simulink model "KUKA_Linear"  (R2020b)
settings: Solver=VariableStepAuto  StartTime=0.0  StopTime=200  RelTol=1e-3
(part 3 of 3)

== matlab function KUKA_Linear/Subsystem/Jacobian//Jacobian_dot//X_dot//X_ddot ==
  data: J output; q1 input; J_dot output; q1_dot input; q2 input; q2_dot input; q3 input; q3_dot input; q4 input; q4_dot input; q1_ddot input; q2_ddot input; q3_ddot input; X_dot output; X_ddot output; q4_ddot input; Theta_dot output; Theta_ddot output
function [J, J_dot, X_dot, X_ddot, Theta_dot, Theta_ddot] = fcn(q1, q1_dot, q2, q2_dot, q3, q3_dot, q4, q4_dot, q1_ddot, q2_ddot, q3_ddot, q4_ddot)

d3 = 0.4;
d5 = 0.39;

%#codegen
theta_1 = q1;
theta_2 = q2;
theta_3 = q3;
theta_4 = q4;

theta_1_dot = q1_dot;
theta_2_dot = q2_dot;
theta_3_dot = q3_dot;
theta_4_dot = q1_dot;

j1 = [  d3*sin(theta_1)*sin(theta_2) - d5*(sin(theta_4)*(cos(theta_1)*sin(theta_3) + cos(theta_2)*cos(theta_3)*sin(theta_1)) - cos(theta_4)*sin(theta_1)*sin(theta_2)), - d5*(cos(theta_1)*cos(theta_2)*cos(theta_4) + cos(theta_1)*cos(theta_3)*sin(theta_2)*sin(theta_4)) - d3*cos(theta_1)*cos(theta_2), -d5*sin(theta_4)*(cos(theta_3)*sin(theta_1) + cos(theta_1)*cos(theta_2)*sin(theta_3)), -d5*(cos(theta_4)*(sin(theta_1)*sin(theta_3) - cos(theta_1)*cos(theta_2)*cos(theta_3)) - cos(theta_1)*sin(theta_2)*sin(theta_4))];
j2 = [- d5*(sin(theta_4)*(sin(theta_1)*sin(theta_3) - cos(theta_1)*cos(theta_2)*cos(theta_3)) + cos(theta_1)*cos(theta_4)*sin(theta_2)) - d3*cos(theta_1)*sin(theta_2), - d5*(cos(theta_2)*cos(theta_4)*sin(theta_1) + cos(theta_3)*sin(theta_1)*sin(theta_2)*sin(theta_4)) - d3*cos(theta_2)*sin(theta_1),  d5*sin(theta_4)*(cos(theta_1)*cos(theta_3) - cos(theta_2)*sin(theta_1)*sin(theta_3)),  d5*(cos(theta_4)*(cos(theta_1)*sin(theta_3) + cos(theta_2)*cos(theta_3)*sin(theta_1)) + sin(theta_1)*sin(theta_2)*sin(theta_4))];
j3 = [                                                                                                                                                               0,                                        - d5*(cos(theta_4)*sin(theta_2) - cos(theta_2)*cos(theta_3)*sin(theta_4)) - d3*sin(theta_2),                                            -d5*sin(theta_2)*sin(theta_3)*sin(theta_4),                                                         -d5*(cos(theta_2)*sin(theta_4) - cos(theta_3)*cos(theta_4)*sin(theta_2))];

Jv = [j1;j2;j3];

j1_dot = [  theta_1_dot*(d5*(sin(theta_4)*(sin(theta_1)*sin(theta_3) - cos(theta_1)*cos(theta_2)*cos(theta_3)) + cos(theta_1)*cos(theta_4)*sin(theta_2)) + d3*cos(theta_1)*sin(theta_2)) + theta_2_dot*(d5*(cos(theta_2)*cos(theta_4)*sin(theta_1) + cos(theta_3)*sin(theta_1)*sin(theta_2)*sin(theta_4)) + d3*cos(theta_2)*sin(theta_1)) - d5*theta_4_dot*(cos(theta_4)*(cos(theta_1)*sin(theta_3) + cos(theta_2)*cos(theta_3)*sin(theta_1)) + sin(theta_1)*sin(theta_2)*sin(theta_4)) - d5*theta_3_dot*sin(theta_4)*(cos(theta_1)*cos(theta_3) - cos(theta_2)*sin(theta_1)*sin(theta_3)), theta_2_dot*(d5*(cos(theta_1)*cos(theta_4)*sin(theta_2) - cos(theta_1)*cos(theta_2)*cos(theta_3)*sin(theta_4)) + d3*cos(theta_1)*sin(theta_2)) + theta_1_dot*(d5*(cos(theta_2)*cos(theta_4)*sin(theta_1) + cos(theta_3)*sin(theta_1)*sin(theta_2)*sin(theta_4)) + d3*cos(theta_2)*sin(theta_1)) + d5*theta_4_dot*(cos(theta_1)*cos(theta_2)*sin(theta_4) - cos(theta_1)*cos(theta_3)*cos(theta_4)*sin(theta_2)) + d5*theta_3_dot*cos(theta_1)*sin(theta_2)*sin(theta_3)*sin(theta_4), d5*theta_3_dot*sin(theta_4)*(sin(theta_1)*sin(theta_3) - cos(theta_1)*cos(theta_2)*cos(theta_3)) - d5*theta_1_dot*sin(theta_4)*(cos(theta_1)*cos(theta_3) - cos(theta_2)*sin(theta_1)*sin(theta_3)) - d5*theta_4_dot*cos(theta_4)*(cos(theta_3)*sin(theta_1) + cos(theta_1)*cos(theta_2)*sin(theta_3)) + d5*theta_2_dot*cos(theta_1)*sin(theta_2)*sin(theta_3)*sin(theta_4), d5*theta_4_dot*(sin(theta_4)*(sin(theta_1)*sin(theta_3) - cos(theta_1)*cos(theta_2)*cos(theta_3)) + cos(theta_1)*cos(theta_4)*sin(theta_2)) - d5*theta_1_dot*(cos(theta_4)*(cos(theta_1)*sin(theta_3) + cos(theta_2)*cos(theta_3)*sin(theta_1)) + sin(theta_1)*sin(theta_2)*sin(theta_4)) + d5*theta_2_dot*(cos(theta_1)*cos(theta_2)*sin(theta_4) - cos(theta_1)*cos(theta_3)*cos(theta_4)*sin(theta_2)) - d5*theta_3_dot*cos(theta_4)*(cos(theta_3)*sin(theta_1) + cos(theta_1)*cos(theta_2)*sin(theta_3))                                                                                                                                                                                                                                                                                                                                                                                                                                                                                                  ];
j2_dot = [- theta_2_dot*(d5*(cos(theta_1)*cos(theta_2)*cos(theta_4) + cos(theta_1)*cos(theta_3)*sin(theta_2)*sin(theta_4)) + d3*cos(theta_1)*cos(theta_2)) - theta_1_dot*(d5*(sin(theta_4)*(cos(theta_1)*sin(theta_3) + cos(theta_2)*cos(theta_3)*sin(theta_1)) - cos(theta_4)*sin(theta_1)*sin(theta_2)) - d3*sin(theta_1)*sin(theta_2)) - d5*theta_4_dot*(cos(theta_4)*(sin(theta_1)*sin(theta_3) - cos(theta_1)*cos(theta_2)*cos(theta_3)) - cos(theta_1)*sin(theta_2)*sin(theta_4)) - d5*theta_3_dot*sin(theta_4)*(cos(theta_3)*sin(theta_1) + cos(theta_1)*cos(theta_2)*sin(theta_3)), theta_2_dot*(d5*(cos(theta_4)*sin(theta_1)*sin(theta_2) - cos(theta_2)*cos(theta_3)*sin(theta_1)*sin(theta_4)) + d3*sin(theta_1)*sin(theta_2)) - theta_1_dot*(d5*(cos(theta_1)*cos(theta_2)*cos(theta_4) + cos(theta_1)*cos(theta_3)*sin(theta_2)*sin(theta_4)) + d3*cos(theta_1)*cos(theta_2)) + d5*theta_4_dot*(cos(theta_2)*sin(theta_1)*sin(theta_4) - cos(theta_3)*cos(theta_4)*sin(theta_1)*sin(theta_2)) + d5*theta_3_dot*sin(theta_1)*sin(theta_2)*sin(theta_3)*sin(theta_4), d5*theta_4_dot*cos(theta_4)*(cos(theta_1)*cos(theta_3) - cos(theta_2)*sin(theta_1)*sin(theta_3)) - d5*theta_1_dot*sin(theta_4)*(cos(theta_3)*sin(theta_1) + cos(theta_1)*cos(theta_2)*sin(theta_3)) - d5*theta_3_dot*sin(theta_4)*(cos(theta_1)*sin(theta_3) + cos(theta_2)*cos(theta_3)*sin(theta_1)) + d5*theta_2_dot*sin(theta_1)*sin(theta_2)*sin(theta_3)*sin(theta_4), d5*theta_2_dot*(cos(theta_2)*sin(theta_1)*sin(theta_4) - cos(theta_3)*cos(theta_4)*sin(theta_1)*sin(theta_2)) - d5*theta_4_dot*(sin(theta_4)*(cos(theta_1)*sin(theta_3) + cos(theta_2)*cos(theta_3)*sin(theta_1)) - cos(theta_4)*sin(theta_1)*sin(theta_2)) - d5*theta_1_dot*(cos(theta_4)*(sin(theta_1)*sin(theta_3) - cos(theta_1)*cos(theta_2)*cos(theta_3)) - cos(theta_1)*sin(theta_2)*sin(theta_4)) + d5*theta_3_dot*cos(theta_4)*(cos(theta_1)*cos(theta_3) - cos(theta_2)*sin(theta_1)*sin(theta_3))                                                                                                                                                                                                                                                                                                                                                                                                                                                                                                  ];
j3_dot = [                                                                                                                                                                                                                                                                                                                                                                                                                                                                                                                                                                               0,                                                                                                                                                                                                                                d5*theta_4_dot*(sin(theta_2)*sin(theta_4) + cos(theta_2)*cos(theta_3)*cos(theta_4)) - theta_2_dot*(d5*(cos(theta_2)*cos(theta_4) + cos(theta_3)*sin(theta_2)*sin(theta_4)) + d3*cos(theta_2)) - d5*theta_3_dot*cos(theta_2)*sin(theta_3)*sin(theta_4),                                                                                                                                                                                                     - d5*theta_2_dot*cos(theta_2)*sin(theta_3)*sin(theta_4) - d5*theta_3_dot*cos(theta_3)*sin(theta_2)*sin(theta_4) - d5*theta_4_dot*cos(theta_4)*sin(theta_2)*sin(theta_3),                                                                                                                                                                                                                                                                            d5*theta_2_dot*(sin(theta_2)*sin(theta_4) + cos(theta_2)*cos(theta_3)*cos(theta_4)) - d5*theta_4_dot*(cos(theta_2)*cos(theta_4) + cos(theta_3)*sin(theta_2)*sin(theta_4)) - d5*theta_3_dot*cos(theta_4)*sin(theta_2)*sin(theta_3)                                                                                                                                                                                                                                                                                                                                                                                                                                                                                                  ];

Jv_dot = [j1_dot;j2_dot;j3_dot];

X_dot = Jv*[q1_dot ; q2_dot ; q3_dot; q4_dot];
X_ddot = Jv_dot*[q1_dot ; q2_dot ; q3_dot; q4_dot] + Jv*[q1_ddot ; q2_ddot ; q3_ddot; q4_ddot];

jw1 = [                                                                                                                                                               0,                                                                                                                       sin(theta_1),                                                            -cos(theta_1)*sin(theta_2),                                                             - cos(theta_3)*sin(theta_1) - cos(theta_1)*cos(theta_2)*sin(theta_3)];
jw2 = [                                                                                                                                                               0,                                                                                                                      -cos(theta_1),                                                            -sin(theta_1)*sin(theta_2),                                                               cos(theta_1)*cos(theta_3) - cos(theta_2)*sin(theta_1)*sin(theta_3)];
jw3 = [                                                                                                                                                               1,                                                                                                                                  0,                                                                          cos(theta_2),                                                                                                       -sin(theta_2)*sin(theta_3)];

Jw = [jw1;jw2;jw3];

jw1_dot = [                                                                                                                                                                                                                                                                                                                                                                                                                                                                                                                                                                               0,                                                                                                                                                                                                                                                                                                                                                                                                                                                             theta_1_dot*cos(theta_1),                                                                                                                                                                                                                                                                                               theta_1_dot*sin(theta_1)*sin(theta_2) - theta_2_dot*cos(theta_1)*cos(theta_2),                                                                                                                                                                                                                                                                                     theta_3_dot*(sin(theta_1)*sin(theta_3) - cos(theta_1)*cos(theta_2)*cos(theta_3)) - theta_1_dot*(cos(theta_1)*cos(theta_3) - cos(theta_2)*sin(theta_1)*sin(theta_3)) + theta_2_dot*cos(theta_1)*sin(theta_2)*sin(theta_3)];
jw2_dot = [                                                                                                                                                                                                                                                                                                                                                                                                                                                                                                                                                                               0,                                                                                                                                                                                                                                                                                                                                                                                                                                                             theta_1_dot*sin(theta_1),                                                                                                                                                                                                                                                                                             - theta_1_dot*cos(theta_1)*sin(theta_2) - theta_2_dot*cos(theta_2)*sin(theta_1),                                                                                                                                                                                                                                                                                     theta_2_dot*sin(theta_1)*sin(theta_2)*sin(theta_3) - theta_3_dot*(cos(theta_1)*sin(theta_3) + cos(theta_2)*cos(theta_3)*sin(theta_1)) - theta_1_dot*(cos(theta_3)*sin(theta_1) + cos(theta_1)*cos(theta_2)*sin(theta_3))];
jw3_dot = [                                                                                                                                                                                                                                                                                                                                                                                                                                                                                                                                                                               0,                                                                                                                                                                                                                                                                                                                                                                                                                                                                                    0,                                                                                                                                                                                                                                                                                                                                                   -theta_2_dot*sin(theta_2),                                                                                                                                                                                                                                                                                                                                                                                                                              - theta_2_dot*cos(theta_2)*sin(theta_3) - theta_3_dot*cos(theta_3)*sin(theta_2)];

Jw_dot = [jw1_dot;jw2_dot;jw3_dot];

Theta_dot = Jw*[q1_dot ; q2_dot ; q3_dot; q4_dot];
Theta_ddot = Jw_dot*[q1_dot ; q2_dot ; q3_dot; q4_dot] + Jw*[q1_ddot ; q2_ddot ; q3_ddot; q4_ddot];

J = [Jv;Jw];
J_dot = [Jv_dot;Jw_dot];

== matlab function KUKA_Linear/POSITION ==
  data: q input; px output; py output; pz output
function [px,py,pz] = fcn(q)
%#codegen

theta_1 = q(1);
theta_2 = q(2);
theta_3 = q(3);
theta_4 = q(4);

d3 = 0.4;
d5 = 0.39;


px = - d5*(sin(theta_4)*(sin(theta_1)*sin(theta_3) - cos(theta_1)*cos(theta_2)*cos(theta_3)) + cos(theta_1)*cos(theta_4)*sin(theta_2)) - d3*cos(theta_1)*sin(theta_2);
py = d5*(sin(theta_4)*(cos(theta_1)*sin(theta_3) + cos(theta_2)*cos(theta_3)*sin(theta_1)) - cos(theta_4)*sin(theta_1)*sin(theta_2)) - d3*sin(theta_1)*sin(theta_2);
pz = d5*(cos(theta_2)*cos(theta_4) + cos(theta_3)*sin(theta_2)*sin(theta_4)) + d3*cos(theta_2);

== matlab function KUKA_Linear/Subsystem/MATLAB Function4 ==
  data: q input; q1 output; q_dot input; q1_dot output; q2 output; q2_dot output; q3 output; q3_dot output; q4 output; q4_dot output; q_ddot input; q1_ddot output; q2_ddot output; q3_ddot output; q4_ddot output
function [q1,q1_dot,q2,q2_dot,q3,q3_dot,q4,q4_dot,q1_ddot,q2_ddot,q3_ddot,q4_ddot] = fcn(q,q_dot,q_ddot)
%#codegen

q1 = q(1);
q2 = q(2);
q3 = q(3);
q4 = q(4);

q1_dot = q_dot(1);
q2_dot = q_dot(2);
q3_dot = q_dot(3);
q4_dot = q_dot(4);

q1_ddot = q_ddot(1);
q2_ddot = q_ddot(2);
q3_ddot = q_ddot(3);
q4_ddot = q_ddot(4);
